simulink model "simulinik_model"  (R2018b)
settings: Solver=VariableStepDiscrete  StartTime=t0  StopTime=tk  RelTol=1e-3
values from neighbouring files (symbols this model uses):
  C = 470*10^(-9)    (= 4.7e-07)    [Lsimem.m]    (also in RLC1.m; RLCanalzia.m; RLCwyjscie.m = [1 0; 0 1; R 0; -R -1]; RLcobwod.m = 2.7e-07)
  L = 220*10^(-6)    (= 0.00022)    [Lsimem.m]    (also in RLC1.m; RLCanalzia.m; RLCwyjscie.m; RLcobwod.m)
  R = 4.7    [Lsimem.m]    (also in RLC1.m; RLCanalzia.m; RLCwyjscie.m; RLcobwod.m)
  ts = 1e-8    (= 1e-08)    [Lsimem.m]    (also in Switchem.m)
undefined symbols (not defined in the file or in its folder): DiscIntNeverNeededParam
settings Model: Creator=user  LastModifiedBy=user

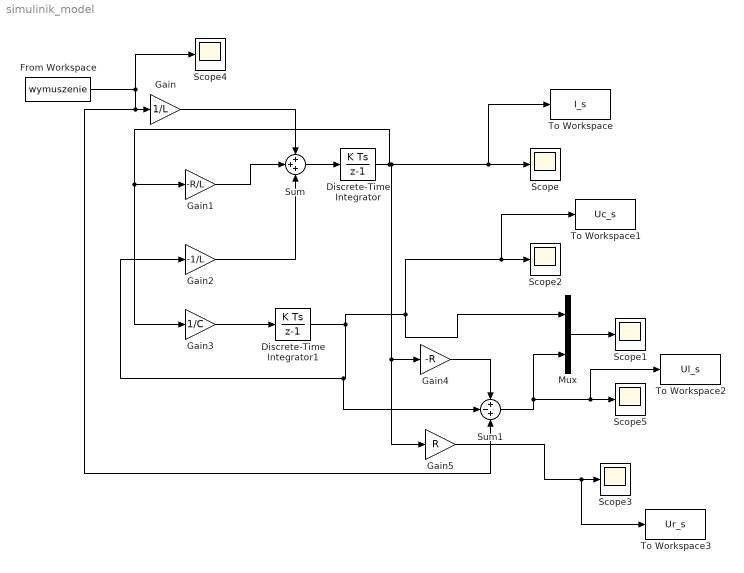
== system simulinik_model ==
  Discrete-Time Integrator : DiscreteIntegrator  SampleTime=ts  ICPrevOutput=DiscIntNeverNeededParam  ICPrevScaledInput=DiscIntNeverNeededParam
  Discrete-Time Integrator1 : DiscreteIntegrator  InitialCondition=ts  SampleTime=-1  ICPrevOutput=DiscIntNeverNeededParam  ICPrevScaledInput=DiscIntNeverNeededParam
  From Workspace : FromWorkspace  VariableName=wymuszenie  SampleTime=ts  OutputAfterFinalValue=Holding final value
  Gain : Gain  Gain=1/L
  Gain1 : Gain  Gain=-R/L
  Gain2 : Gain  Gain=-1/L
  Gain3 : Gain  Gain=1/C
  Gain4 : Gain  Gain=-R
  Gain5 : Gain  Gain=R
  Mux : Mux  Inputs=2
  Scope{,1..5} (6 alike) : Scope
  Sum : Sum  Inputs=+++
  Sum1 : Sum  Inputs=+-+
  To Workspace : ToWorkspace  VariableName=I_s  SampleTime=-1
      settings: Save2DSignal=2-D array (concatenate along first dimension)
  To Workspace1 : ToWorkspace  VariableName=Uc_s  SampleTime=-1
      settings: Save2DSignal=2-D array (concatenate along first dimension)
  To Workspace2 : ToWorkspace  VariableName=Ul_s  SampleTime=-1
      settings: Save2DSignal=2-D array (concatenate along first dimension)
  To Workspace3 : ToWorkspace  VariableName=Ur_s  SampleTime=-1
      settings: Save2DSignal=2-D array (concatenate along first dimension)
  wires:
  From Workspace/1 -> Sum1/3, Gain/1, Scope4/1
  Gain/1 -> Sum/1
  Gain1/1 -> Sum/2
  Gain2/1 -> Sum/3
  Sum/1 -> Discrete-Time Integrator/1
  Discrete-Time Integrator/1 -> Gain5/1, Gain4/1, To Workspace/1, Scope/1, Gain3/1, Gain1/1
  Gain3/1 -> Discrete-Time Integrator1/1
  Discrete-Time Integrator1/1 -> Mux/1, To Workspace1/1, Scope2/1, Sum1/2, Gain2/1
  Gain4/1 -> Sum1/1
  Gain5/1 -> To Workspace3/1, Scope3/1
  Sum1/1 -> To Workspace2/1, Scope5/1, Mux/2
  Mux/1 -> Scope1/1
